simulink library "FlexBeamElement_MS2G_Lib"  (R2016a)
settings: Solver=ode45  StartTime=0.0  StopTime=10.0  RelTol=1e-3
undefined symbols (not defined in the file): b, beam_length, beam_wall, beam_width, bending_stiffness, Damping, density, Extr_Data_Box, kbendingx, kbendingy, kelongz, ktwistz, matDamping, num_elem, numelem, rho, shearM, X, Y, youngsM, Z
libraries: sm_lib x335, nesl_utility x64, FlexBeamElement_MS2G_Lib x1
(part 2 of 10)

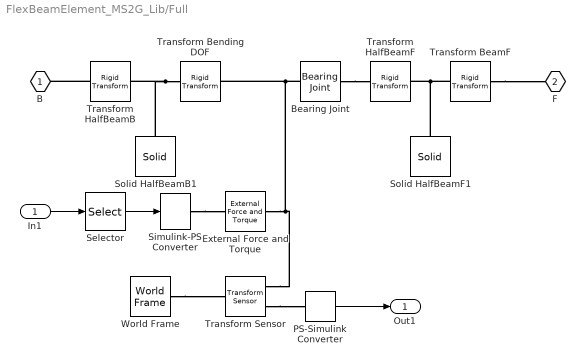
== system FlexBeamElement_MS2G_Lib/Full ==
  In1 : Inport
  " Transform Bending DOF" : sm_lib/Frames and Transforms/Rigid Transform  TranslationMethod=StandardAxis  TranslationLengthUnit=m  TranslationStandardAxis=+Z  TranslationStandardOffset=length/4  TranslationCartesianOffset=[0 0 0]  TranslationROffset=0  TranslationROffsetUnits=m  TranslationZOffset=0  TranslationZOffsetUnits=m  TranslationThetaOffset=0  TranslationThetaOffsetUnits=deg  RotationMethod=None  RotationAngleUnits=deg  RotationStandardAxis=+Y  RotationAngle=90  RotationArbitraryAxis=[0 0 1]  FollAlignAxisA=+X  BaseAlignAxisA=+Y  FollAlignAxisB=+Y  BaseAlignAxisB=+Z  RotationSequenceAxes=FollowerAxes  RotationSequence=XYX  RotationSequenceAngles=[0 0 0]  RotationSequenceAnglesUnits=deg  RotationMatrix=[1 0 0; 0 1 0; 0 0 1]
  " Transform BeamF" : sm_lib/Frames and Transforms/Rigid Transform  TranslationMethod=StandardAxis  TranslationLengthUnit=m  TranslationStandardAxis=+Z  TranslationStandardOffset=length/4  TranslationCartesianOffset=[0 0 0]  TranslationROffset=0  TranslationROffsetUnits=m  TranslationZOffset=0  TranslationZOffsetUnits=m  TranslationThetaOffset=0  TranslationThetaOffsetUnits=deg  RotationMethod=None  RotationAngleUnits=deg  RotationStandardAxis=+Z  RotationAngle=0  RotationArbitraryAxis=[0 0 1]  FollAlignAxisA=+X  BaseAlignAxisA=+Y  FollAlignAxisB=+Y  BaseAlignAxisB=+Z  RotationSequenceAxes=FollowerAxes  RotationSequence=XYX  RotationSequenceAngles=[0 0 0]  RotationSequenceAnglesUnits=deg  RotationMatrix=[1 0 0; 0 1 0; 0 0 1]
  Bearing Joint : sm_lib/Joints/Bearing Joint  SenseConstraintForce=off  SenseConstraintForceX=off  SenseConstraintForceY=off  SenseConstraintForceZ=off  SenseConstraintTorque=off  SenseConstraintTorqueX=off  SenseConstraintTorqueY=off  SenseConstraintTorqueZ=off  SenseTotalForce=off  SenseTotalForceX=off  SenseTotalForceY=off  SenseTotalForceZ=off  SenseTotalTorque=off  SenseTotalTorqueX=off  SenseTotalTorqueY=off  SenseTotalTorqueZ=off  CompositeWrenchDir=FollowerOnBase  CompositeWrenchFrame=BaseFrame  PzEquilibriumPosition=0  PzEquilibriumPositionUnits=m  PzSpringStiffness=kelongz  PzSpringStiffnessUnits=N/m  PzDampingCoefficient=b  PzDampingCoefficientUnits=N/(m/s)  PzTorqueActuationMode=NoTorque  PzMotionActuationMode=ComputedMotion  PzSensePosition=off  PzSenseVelocity=off  PzSenseAcceleration=off  PzSenseTorqueForce=off  PzPositionTargetSpecify=off  PzPositionTargetPriority=High  PzPositionTargetValue=0  PzPositionTargetValueUnits=m  PzVelocityTargetSpecify=off  PzVelocityTargetPriority=High  PzVelocityTargetValue=0  PzVelocityTargetValueUnits=m/s  RxEquilibriumPosition=0  RxEquilibriumPositionUnits=deg  RxSpringStiffness=kbendingx  RxSpringStiffnessUnits=N*m/rad  RxDampingCoefficient=b  RxDampingCoefficientUnits=N*m/(rad/s)  RxTorqueActuationMode=NoTorque  RxMotionActuationMode=ComputedMotion  RxSensePosition=off  RxSenseVelocity=off  RxSenseAcceleration=off  RxSenseTorqueForce=off  RxPositionTargetSpecify=off  RxPositionTargetPriority=High  RxPositionTargetValue=0  RxPositionTargetValueUnits=deg  RxVelocityTargetSpecify=off  RxVelocityTargetPriority=High  RxVelocityTargetValue=0  RxVelocityTargetValueUnits=deg/s  RyEquilibriumPosition=0  RyEquilibriumPositionUnits=deg  RySpringStiffness=kbendingy  RySpringStiffnessUnits=N*m/rad  RyDampingCoefficient=b  RyDampingCoefficientUnits=N*m/(rad/s)  RyTorqueActuationMode=NoTorque  RyMotionActuationMode=ComputedMotion  RySensePosition=off  RySenseVelocity=off  RySenseAcceleration=off  RySenseTorqueForce=off  RyPositionTargetSpecify=off  RyPositionTargetPriority=High  RyPositionTargetValue=0  RyPositionTargetValueUnits=deg  RyVelocityTargetSpecify=off  RyVelocityTargetPriority=High  RyVelocityTargetValue=0  RyVelocityTargetValueUnits=deg/s  RzEquilibriumPosition=0  RzEquilibriumPositionUnits=deg  RzSpringStiffness=ktwistz  RzSpringStiffnessUnits=N*m/rad  RzDampingCoefficient=b  RzDampingCoefficientUnits=N*m/(rad/s)  RzTorqueActuationMode=NoTorque  RzMotionActuationMode=ComputedMotion  RzSensePosition=off  RzSenseVelocity=off  RzSenseAcceleration=off  RzSenseTorqueForce=off  RzPositionTargetSpecify=off  RzPositionTargetPriority=High  RzPositionTargetValue=0  RzPositionTargetValueUnits=deg  RzVelocityTargetSpecify=off  RzVelocityTargetPriority=High  RzVelocityTargetValue=0  RzVelocityTargetValueUnits=deg/s
  External Force and Torque : sm_lib/Forces and Torques/External Force and Torque  ForceResolutionFrame=AttachedFrame  EnableForceX=off  EnableForceY=off  EnableForceZ=off  EnableForce=on  TorqueResolutionFrame=AttachedFrame  EnableTorqueX=off  EnableTorqueY=off  EnableTorqueZ=off  EnableTorque=off
  PS-Simulink Converter : nesl_utility/PS-Simulink Converter  PhysicalDomain=network_engine_domain  SubClassName=ps_output  LeftPortType=input  RightPortType=output  PseudoPeriodic=off  Frequencies=[]  Unit=1  AffineConversion=off
  Selector : Selector  InputPortWidth=numelem*3  IndexOptions=Index vector (dialog)  Indices=[1 3]  OutputSizes=1
  Simulink-PS Converter : nesl_utility/Simulink-PS Converter  PhysicalDomain=network_engine_domain  SubClassName=ps_input  LeftPortType=input  RightPortType=output  PseudoPeriodic=off  Frequencies=[]  NoiseDistribution=none  NoiseParameters=[]  Unit=1  AffineConversion=off  InputFiltering=off  SimscapeFilterOrder=1  InputFilterTimeConstant=0.001  UdotUserProvided=1
  Solid HalfBeamB1 : sm_lib/Body Elements/Solid  InertiaType=CalculateFromGeometry  Mass=1  MassUnits=kg  CenterOfMass=[0 0 0]  CenterOfMassUnits=m  MomentsOfInertia=[1 1 1]  MomentsOfInertiaUnits=kg*m^2  ProductsOfInertia=[0 0 0]  ProductsOfInertiaUnits=kg*m^2  DensityBased=on  Density=rho  DensityUnits=kg/(m^3)  DoExposeReferenceFrame=on  SerializedFrames=<Frames/>  GraphicType=FromGeometry  MarkerShape=Sphere  MarkerSize=10  MarkerSizeUnits=m  GraphicVisPropType=SimpleVisualProperties  GraphicDiffuseColor=[0.5 0.5 0.5]  GraphicSpecularColor=[0.5 0.5 0.5 1.0]  GraphicAmbientColor=[0.15 0.15 0.15 1.0]  GraphicEmissiveColor=[0.0 0.0 0.0 1.0]  GraphicShininess=75  GraphicOpacity=1.0  GeometryShape=GeneralExtrusion  RectangleSize=[1 1]  RectangleSizeUnits=m  BrickDimensions=[1 1 1]  BrickDimensionUnits=m  CylinderRadius=1  CylinderRadiusUnits=m  CylinderLength=1  CylinderLengthUnits=m  SphereRadius=1  SphereRadiusUnits=m  EllipsoidRadii=[1 1 1]  EllipsoidRadiiUnits=m  ExtrusionCrossSection=Extr_Data_Box(beam_width,beam_width-2*beam_wall,beam_width,beam_width-2*beam_wall)  ExtrusionCrossSectionUnits=m  ExtrusionLength=length/2  ExtrusionLengthUnits=m  PolygonNumSides=3  PolygonOuterRadius=1  PolygonOuterRadiusUnits=m  ExtGeomFileType=STL  ExtGeomFileUnits=m  RevolutionCrossSection=[1 1; 1 -1; 2 -1; 2 1]  RevolutionCrossSectionUnits=m  RevolutionExtent=Full  RevolutionAngle=180  RevolutionAngleUnits=deg
  Solid HalfBeamF1 : sm_lib/Body Elements/Solid  InertiaType=CalculateFromGeometry  Mass=1  MassUnits=kg  CenterOfMass=[0 0 0]  CenterOfMassUnits=m  MomentsOfInertia=[1 1 1]  MomentsOfInertiaUnits=kg*m^2  ProductsOfInertia=[0 0 0]  ProductsOfInertiaUnits=kg*m^2  DensityBased=on  Density=rho  DensityUnits=kg/(m^3)  DoExposeReferenceFrame=on  SerializedFrames=<Frames/>  GraphicType=FromGeometry  MarkerShape=Sphere  MarkerSize=10  MarkerSizeUnits=m  GraphicVisPropType=SimpleVisualProperties  GraphicDiffuseColor=[0.5 0.5 0.5]  GraphicSpecularColor=[0.5 0.5 0.5 1.0]  GraphicAmbientColor=[0.15 0.15 0.15 1.0]  GraphicEmissiveColor=[0.0 0.0 0.0 1.0]  GraphicShininess=75  GraphicOpacity=1.0  GeometryShape=GeneralExtrusion  RectangleSize=[1 1]  RectangleSizeUnits=m  BrickDimensions=[1 1 1]  BrickDimensionUnits=m  CylinderRadius=1  CylinderRadiusUnits=m  CylinderLength=1  CylinderLengthUnits=m  SphereRadius=1  SphereRadiusUnits=m  EllipsoidRadii=[1 1 1]  EllipsoidRadiiUnits=m  ExtrusionCrossSection=Extr_Data_Box(beam_width,beam_width-2*beam_wall,beam_width,beam_width-2*beam_wall)  ExtrusionCrossSectionUnits=m  ExtrusionLength=length/2  ExtrusionLengthUnits=m  PolygonNumSides=3  PolygonOuterRadius=1  PolygonOuterRadiusUnits=m  ExtGeomFileType=STL  ExtGeomFileUnits=m  RevolutionCrossSection=[1 1; 1 -1; 2 -1; 2 1]  RevolutionCrossSectionUnits=m  RevolutionExtent=Full  RevolutionAngle=180  RevolutionAngleUnits=deg
  Transform HalfBeamB : sm_lib/Frames and Transforms/Rigid Transform  TranslationMethod=StandardAxis  TranslationLengthUnit=m  TranslationStandardAxis=+Z  TranslationStandardOffset=length/4  TranslationCartesianOffset=[0 0 0]  TranslationROffset=0  TranslationROffsetUnits=m  TranslationZOffset=0  TranslationZOffsetUnits=m  TranslationThetaOffset=0  TranslationThetaOffsetUnits=deg  RotationMethod=None  RotationAngleUnits=deg  RotationStandardAxis=+Z  RotationAngle=0  RotationArbitraryAxis=[0 0 1]  FollAlignAxisA=+X  BaseAlignAxisA=+Y  FollAlignAxisB=+Y  BaseAlignAxisB=+Z  RotationSequenceAxes=FollowerAxes  RotationSequence=XYX  RotationSequenceAngles=[0 0 0]  RotationSequenceAnglesUnits=deg  RotationMatrix=[1 0 0; 0 1 0; 0 0 1]
  Transform HalfBeamF : sm_lib/Frames and Transforms/Rigid Transform  TranslationMethod=StandardAxis  TranslationLengthUnit=m  TranslationStandardAxis=+Z  TranslationStandardOffset=-length/4  TranslationCartesianOffset=[0 0 0]  TranslationROffset=0  TranslationROffsetUnits=m  TranslationZOffset=0  TranslationZOffsetUnits=m  TranslationThetaOffset=0  TranslationThetaOffsetUnits=deg  RotationMethod=None  RotationAngleUnits=deg  RotationStandardAxis=+Y  RotationAngle=90  RotationArbitraryAxis=[0 0 1]  FollAlignAxisA=+X  BaseAlignAxisA=+Y  FollAlignAxisB=+Y  BaseAlignAxisB=+Z  RotationSequenceAxes=FollowerAxes  RotationSequence=XYX  RotationSequenceAngles=[0 0 0]  RotationSequenceAnglesUnits=deg  RotationMatrix=[1 0 0; 0 1 0; 0 0 1]
  Transform Sensor : sm_lib/Frames and Transforms/Transform Sensor  MeasurementFrame=World  SenseAngle=off  SenseAxis=off  SenseAngle1=off  SenseAngle2=off  SenseAngle3=off  SenseQ=off  SenseR=off  SenseOmegaX=off  SenseOmegaY=off  SenseOmegaZ=on  SenseOmega1=off  SenseOmega2=off  SenseOmega3=off  SenseQDot=off  SenseRDot=off  SenseAlphaX=off  SenseAlphaY=off  SenseAlphaZ=off  SenseAlpha1=off  SenseAlpha2=off  SenseAlpha3=off  SenseQDDot=off  SenseRDDot=off  SenseX=off  SenseY=off  SenseZ=off  SenseRad=off  SenseAzim=off  SenseDist=off  SenseInc=off  SenseXDot=off  SenseYDot=off  SenseZDot=off  SenseRadDot=off  SenseAzimDot=off  SenseDistDot=off  SenseIncDot=off  SenseXDDot=off  SenseYDDot=off  SenseZDDot=off  SenseRadDDot=off  SenseAzimDDot=off  SenseDistDDot=off  SenseIncDDot=off
  World Frame : sm_lib/Frames and Transforms/World Frame
  B : PMIOPort  Port=1  Side=Left
  F : PMIOPort  Port=2  Side=Right
  Out1 : Outport
  wires:
  In1/1 -> Selector/1
  Selector/1 -> Simulink-PS Converter/1
  PS-Simulink Converter/1 -> Out1/1
  connections:
  External Force and Torque/RConn1 -- Transform Sensor/RConn1 -- " Transform Bending DOF"/RConn1 -- Bearing Joint/LConn1
  Bearing Joint/RConn1 -- Transform HalfBeamF/RConn1
  " Transform Bending DOF"/LConn1 -- Transform HalfBeamB/RConn1 -- Solid HalfBeamB1/RConn1
  Solid HalfBeamF1/RConn1 -- " Transform BeamF"/LConn1 -- Transform HalfBeamF/LConn1
  Transform HalfBeamB/LConn1 -- B/RConn1
  " Transform BeamF"/RConn1 -- F/RConn1
  Simulink-PS Converter/RConn1 -- External Force and Torque/LConn1
  World Frame/RConn1 -- Transform Sensor/LConn1
  Transform Sensor/RConn2 -- PS-Simulink Converter/LConn1

== system FlexBeamElement_MS2G_Lib/Flex_Body/Flex_Elem_1 ==
  In1 : Inport
  Full : Subsystem  mask{length=length, rho=rho, beam_width=beam_width, beam_wall=beam_wall, kbendingx=kbendingx, kbendingy=kbendingy, kbendingz=ktwistz, kelongz=kelongz, b=b}
      mask prompts: length "Beam Length (m)"; rho "Material Density (kg/(m^3)"; beam_width "Beam Width & Height (m)"; beam_wall "Beam Wall Thickness (m)"; kbendingx "Bending Spring Constant about X(Nm/rad)"; kbendingy "Bending Spring Constant about Y(Nm/rad)"; kbendingz "Twist Spring Constant about Z(Nm/rad)"; kelongz "Elongation Spring Constant about Z(N/m)"; b "Damping Constant (Nm/rad.s)"
  B : PMIOPort  Port=1  Side=Left
  F : PMIOPort  Port=2  Side=Right
  Out1 : Outport
  wires:
  In1/1 -> Full/1(In1)
  Full/1(Out1) -> Out1/1
  connections:
  Full/LConn1 -- B/RConn1
  Full/RConn1 -- F/RConn1

== system FlexBeamElement_MS2G_Lib/Flex_Body/Flex_Elem_10 ==
  In1 : Inport
  Full : Subsystem  mask{length=length, rho=rho, beam_width=beam_width, beam_wall=beam_wall, kbendingx=kbendingx, kbendingy=kbendingy, kbendingz=ktwistz, kelongz=kelongz, b=b}
      mask prompts: length "Beam Length (m)"; rho "Material Density (kg/(m^3)"; beam_width "Beam Width & Height (m)"; beam_wall "Beam Wall Thickness (m)"; kbendingx "Bending Spring Constant about X(Nm/rad)"; kbendingy "Bending Spring Constant about Y(Nm/rad)"; kbendingz "Twist Spring Constant about Z(Nm/rad)"; kelongz "Elongation Spring Constant about Z(N/m)"; b "Damping Constant (Nm/rad.s)"
  B : PMIOPort  Port=1  Side=Left
  F : PMIOPort  Port=2  Side=Right
  Out1 : Outport
  wires:
  In1/1 -> Full/1(In1)
  Full/1(Out1) -> Out1/1
  connections:
  Full/LConn1 -- B/RConn1
  Full/RConn1 -- F/RConn1

== system FlexBeamElement_MS2G_Lib/Flex_Body/Flex_Elem_11 ==
  In1 : Inport
  Full : Subsystem  mask{length=length, rho=rho, beam_width=beam_width, beam_wall=beam_wall, kbendingx=kbendingx, kbendingy=kbendingy, kbendingz=ktwistz, kelongz=kelongz, b=b}
      mask prompts: length "Beam Length (m)"; rho "Material Density (kg/(m^3)"; beam_width "Beam Width & Height (m)"; beam_wall "Beam Wall Thickness (m)"; kbendingx "Bending Spring Constant about X(Nm/rad)"; kbendingy "Bending Spring Constant about Y(Nm/rad)"; kbendingz "Twist Spring Constant about Z(Nm/rad)"; kelongz "Elongation Spring Constant about Z(N/m)"; b "Damping Constant (Nm/rad.s)"
  B : PMIOPort  Port=1  Side=Left
  F : PMIOPort  Port=2  Side=Right
  Out1 : Outport
  wires:
  In1/1 -> Full/1(In1)
  Full/1(Out1) -> Out1/1
  connections:
  Full/LConn1 -- B/RConn1
  Full/RConn1 -- F/RConn1

== system FlexBeamElement_MS2G_Lib/Flex_Body/Flex_Elem_12 ==
  In1 : Inport
  Full : Subsystem  mask{length=length, rho=rho, beam_width=beam_width, beam_wall=beam_wall, kbendingx=kbendingx, kbendingy=kbendingy, kbendingz=ktwistz, kelongz=kelongz, b=b}
      mask prompts: length "Beam Length (m)"; rho "Material Density (kg/(m^3)"; beam_width "Beam Width & Height (m)"; beam_wall "Beam Wall Thickness (m)"; kbendingx "Bending Spring Constant about X(Nm/rad)"; kbendingy "Bending Spring Constant about Y(Nm/rad)"; kbendingz "Twist Spring Constant about Z(Nm/rad)"; kelongz "Elongation Spring Constant about Z(N/m)"; b "Damping Constant (Nm/rad.s)"
  B : PMIOPort  Port=1  Side=Left
  F : PMIOPort  Port=2  Side=Right
  Out1 : Outport
  wires:
  In1/1 -> Full/1(In1)
  Full/1(Out1) -> Out1/1
  connections:
  Full/LConn1 -- B/RConn1
  Full/RConn1 -- F/RConn1

== system FlexBeamElement_MS2G_Lib/Flex_Body/Flex_Elem_13 ==
  In1 : Inport
  Full : Subsystem  mask{length=length, rho=rho, beam_width=beam_width, beam_wall=beam_wall, kbendingx=kbendingx, kbendingy=kbendingy, kbendingz=ktwistz, kelongz=kelongz, b=b}
      mask prompts: length "Beam Length (m)"; rho "Material Density (kg/(m^3)"; beam_width "Beam Width & Height (m)"; beam_wall "Beam Wall Thickness (m)"; kbendingx "Bending Spring Constant about X(Nm/rad)"; kbendingy "Bending Spring Constant about Y(Nm/rad)"; kbendingz "Twist Spring Constant about Z(Nm/rad)"; kelongz "Elongation Spring Constant about Z(N/m)"; b "Damping Constant (Nm/rad.s)"
  B : PMIOPort  Port=1  Side=Left
  F : PMIOPort  Port=2  Side=Right
  Out1 : Outport
  wires:
  In1/1 -> Full/1(In1)
  Full/1(Out1) -> Out1/1
  connections:
  Full/LConn1 -- B/RConn1
  Full/RConn1 -- F/RConn1

== system FlexBeamElement_MS2G_Lib/Flex_Body/Flex_Elem_14 ==
  In1 : Inport
  Full : Subsystem  mask{length=length, rho=rho, beam_width=beam_width, beam_wall=beam_wall, kbendingx=kbendingx, kbendingy=kbendingy, kbendingz=ktwistz, kelongz=kelongz, b=b}
      mask prompts: length "Beam Length (m)"; rho "Material Density (kg/(m^3)"; beam_width "Beam Width & Height (m)"; beam_wall "Beam Wall Thickness (m)"; kbendingx "Bending Spring Constant about X(Nm/rad)"; kbendingy "Bending Spring Constant about Y(Nm/rad)"; kbendingz "Twist Spring Constant about Z(Nm/rad)"; kelongz "Elongation Spring Constant about Z(N/m)"; b "Damping Constant (Nm/rad.s)"
  B : PMIOPort  Port=1  Side=Left
  F : PMIOPort  Port=2  Side=Right
  Out1 : Outport
  wires:
  In1/1 -> Full/1(In1)
  Full/1(Out1) -> Out1/1
  connections:
  Full/LConn1 -- B/RConn1
  Full/RConn1 -- F/RConn1

== system FlexBeamElement_MS2G_Lib/Flex_Body/Flex_Elem_15 ==
  In1 : Inport
  Full : Subsystem  mask{length=length, rho=rho, beam_width=beam_width, beam_wall=beam_wall, kbendingx=kbendingx, kbendingy=kbendingy, kbendingz=ktwistz, kelongz=kelongz, b=b}
      mask prompts: length "Beam Length (m)"; rho "Material Density (kg/(m^3)"; beam_width "Beam Width & Height (m)"; beam_wall "Beam Wall Thickness (m)"; kbendingx "Bending Spring Constant about X(Nm/rad)"; kbendingy "Bending Spring Constant about Y(Nm/rad)"; kbendingz "Twist Spring Constant about Z(Nm/rad)"; kelongz "Elongation Spring Constant about Z(N/m)"; b "Damping Constant (Nm/rad.s)"
  B : PMIOPort  Port=1  Side=Left
  F : PMIOPort  Port=2  Side=Right
  Out1 : Outport
  wires:
  In1/1 -> Full/1(In1)
  Full/1(Out1) -> Out1/1
  connections:
  Full/LConn1 -- B/RConn1
  Full/RConn1 -- F/RConn1

== system FlexBeamElement_MS2G_Lib/Flex_Body/Flex_Elem_16 ==
  In1 : Inport
  Full : Subsystem  mask{length=length, rho=rho, beam_width=beam_width, beam_wall=beam_wall, kbendingx=kbendingx, kbendingy=kbendingy, kbendingz=ktwistz, kelongz=kelongz, b=b}
      mask prompts: length "Beam Length (m)"; rho "Material Density (kg/(m^3)"; beam_width "Beam Width & Height (m)"; beam_wall "Beam Wall Thickness (m)"; kbendingx "Bending Spring Constant about X(Nm/rad)"; kbendingy "Bending Spring Constant about Y(Nm/rad)"; kbendingz "Twist Spring Constant about Z(Nm/rad)"; kelongz "Elongation Spring Constant about Z(N/m)"; b "Damping Constant (Nm/rad.s)"
  B : PMIOPort  Port=1  Side=Left
  F : PMIOPort  Port=2  Side=Right
  Out1 : Outport
  wires:
  In1/1 -> Full/1(In1)
  Full/1(Out1) -> Out1/1
  connections:
  Full/LConn1 -- B/RConn1
  Full/RConn1 -- F/RConn1

== system FlexBeamElement_MS2G_Lib/Flex_Body/Flex_Elem_17 ==
  In1 : Inport
  Full : Subsystem  mask{length=length, rho=rho, beam_width=beam_width, beam_wall=beam_wall, kbendingx=kbendingx, kbendingy=kbendingy, kbendingz=ktwistz, kelongz=kelongz, b=b}
      mask prompts: length "Beam Length (m)"; rho "Material Density (kg/(m^3)"; beam_width "Beam Width & Height (m)"; beam_wall "Beam Wall Thickness (m)"; kbendingx "Bending Spring Constant about X(Nm/rad)"; kbendingy "Bending Spring Constant about Y(Nm/rad)"; kbendingz "Twist Spring Constant about Z(Nm/rad)"; kelongz "Elongation Spring Constant about Z(N/m)"; b "Damping Constant (Nm/rad.s)"
  B : PMIOPort  Port=1  Side=Left
  F : PMIOPort  Port=2  Side=Right
  Out1 : Outport
  wires:
  In1/1 -> Full/1(In1)
  Full/1(Out1) -> Out1/1
  connections:
  Full/LConn1 -- B/RConn1
  Full/RConn1 -- F/RConn1

== system FlexBeamElement_MS2G_Lib/Flex_Body/Flex_Elem_18 ==
  In1 : Inport
  Full : Subsystem  mask{length=length, rho=rho, beam_width=beam_width, beam_wall=beam_wall, kbendingx=kbendingx, kbendingy=kbendingy, kbendingz=ktwistz, kelongz=kelongz, b=b}
      mask prompts: length "Beam Length (m)"; rho "Material Density (kg/(m^3)"; beam_width "Beam Width & Height (m)"; beam_wall "Beam Wall Thickness (m)"; kbendingx "Bending Spring Constant about X(Nm/rad)"; kbendingy "Bending Spring Constant about Y(Nm/rad)"; kbendingz "Twist Spring Constant about Z(Nm/rad)"; kelongz "Elongation Spring Constant about Z(N/m)"; b "Damping Constant (Nm/rad.s)"
  B : PMIOPort  Port=1  Side=Left
  F : PMIOPort  Port=2  Side=Right
  Out1 : Outport
  wires:
  In1/1 -> Full/1(In1)
  Full/1(Out1) -> Out1/1
  connections:
  Full/LConn1 -- B/RConn1
  Full/RConn1 -- F/RConn1

== system FlexBeamElement_MS2G_Lib/Flex_Body/Flex_Elem_19 ==
  In1 : Inport
  Full : Subsystem  mask{length=length, rho=rho, beam_width=beam_width, beam_wall=beam_wall, kbendingx=kbendingx, kbendingy=kbendingy, kbendingz=ktwistz, kelongz=kelongz, b=b}
      mask prompts: length "Beam Length (m)"; rho "Material Density (kg/(m^3)"; beam_width "Beam Width & Height (m)"; beam_wall "Beam Wall Thickness (m)"; kbendingx "Bending Spring Constant about X(Nm/rad)"; kbendingy "Bending Spring Constant about Y(Nm/rad)"; kbendingz "Twist Spring Constant about Z(Nm/rad)"; kelongz "Elongation Spring Constant about Z(N/m)"; b "Damping Constant (Nm/rad.s)"
  B : PMIOPort  Port=1  Side=Left
  F : PMIOPort  Port=2  Side=Right
  Out1 : Outport
  wires:
  In1/1 -> Full/1(In1)
  Full/1(Out1) -> Out1/1
  connections:
  Full/LConn1 -- B/RConn1
  Full/RConn1 -- F/RConn1

== system FlexBeamElement_MS2G_Lib/Flex_Body/Flex_Elem_2 ==
  In1 : Inport
  Full : Subsystem  mask{length=length, rho=rho, beam_width=beam_width, beam_wall=beam_wall, kbendingx=kbendingx, kbendingy=kbendingy, kbendingz=ktwistz, kelongz=kelongz, b=b}
      mask prompts: length "Beam Length (m)"; rho "Material Density (kg/(m^3)"; beam_width "Beam Width & Height (m)"; beam_wall "Beam Wall Thickness (m)"; kbendingx "Bending Spring Constant about X(Nm/rad)"; kbendingy "Bending Spring Constant about Y(Nm/rad)"; kbendingz "Twist Spring Constant about Z(Nm/rad)"; kelongz "Elongation Spring Constant about Z(N/m)"; b "Damping Constant (Nm/rad.s)"
  B : PMIOPort  Port=1  Side=Left
  F : PMIOPort  Port=2  Side=Right
  Out1 : Outport
  wires:
  In1/1 -> Full/1(In1)
  Full/1(Out1) -> Out1/1
  connections:
  Full/LConn1 -- B/RConn1
  Full/RConn1 -- F/RConn1

== system FlexBeamElement_MS2G_Lib/Flex_Body/Flex_Elem_20 ==
  In1 : Inport
  Full : Subsystem  mask{length=length, rho=rho, beam_width=beam_width, beam_wall=beam_wall, kbendingx=kbendingx, kbendingy=kbendingy, kbendingz=ktwistz, kelongz=kelongz, b=b}
      mask prompts: length "Beam Length (m)"; rho "Material Density (kg/(m^3)"; beam_width "Beam Width & Height (m)"; beam_wall "Beam Wall Thickness (m)"; kbendingx "Bending Spring Constant about X(Nm/rad)"; kbendingy "Bending Spring Constant about Y(Nm/rad)"; kbendingz "Twist Spring Constant about Z(Nm/rad)"; kelongz "Elongation Spring Constant about Z(N/m)"; b "Damping Constant (Nm/rad.s)"
  B : PMIOPort  Port=1  Side=Left
  F : PMIOPort  Port=2  Side=Right
  Out1 : Outport
  wires:
  In1/1 -> Full/1(In1)
  Full/1(Out1) -> Out1/1
  connections:
  Full/LConn1 -- B/RConn1
  Full/RConn1 -- F/RConn1

== system FlexBeamElement_MS2G_Lib/Flex_Body/Flex_Elem_21 ==
  In1 : Inport
  Full : Subsystem  mask{length=length, rho=rho, beam_width=beam_width, beam_wall=beam_wall, kbendingx=kbendingx, kbendingy=kbendingy, kbendingz=ktwistz, kelongz=kelongz, b=b}
      mask prompts: length "Beam Length (m)"; rho "Material Density (kg/(m^3)"; beam_width "Beam Width & Height (m)"; beam_wall "Beam Wall Thickness (m)"; kbendingx "Bending Spring Constant about X(Nm/rad)"; kbendingy "Bending Spring Constant about Y(Nm/rad)"; kbendingz "Twist Spring Constant about Z(Nm/rad)"; kelongz "Elongation Spring Constant about Z(N/m)"; b "Damping Constant (Nm/rad.s)"
  B : PMIOPort  Port=1  Side=Left
  F : PMIOPort  Port=2  Side=Right
  Out1 : Outport
  wires:
  In1/1 -> Full/1(In1)
  Full/1(Out1) -> Out1/1
  connections:
  Full/LConn1 -- B/RConn1
  Full/RConn1 -- F/RConn1

== system FlexBeamElement_MS2G_Lib/Flex_Body/Flex_Elem_22 ==
  In1 : Inport
  Full : Subsystem  mask{length=length, rho=rho, beam_width=beam_width, beam_wall=beam_wall, kbendingx=kbendingx, kbendingy=kbendingy, kbendingz=ktwistz, kelongz=kelongz, b=b}
      mask prompts: length "Beam Length (m)"; rho "Material Density (kg/(m^3)"; beam_width "Beam Width & Height (m)"; beam_wall "Beam Wall Thickness (m)"; kbendingx "Bending Spring Constant about X(Nm/rad)"; kbendingy "Bending Spring Constant about Y(Nm/rad)"; kbendingz "Twist Spring Constant about Z(Nm/rad)"; kelongz "Elongation Spring Constant about Z(N/m)"; b "Damping Constant (Nm/rad.s)"
  B : PMIOPort  Port=1  Side=Left
  F : PMIOPort  Port=2  Side=Right
  Out1 : Outport
  wires:
  In1/1 -> Full/1(In1)
  Full/1(Out1) -> Out1/1
  connections:
  Full/LConn1 -- B/RConn1
  Full/RConn1 -- F/RConn1

== system FlexBeamElement_MS2G_Lib/Flex_Body/Flex_Elem_23 ==
  In1 : Inport
  Full : Subsystem  mask{length=length, rho=rho, beam_width=beam_width, beam_wall=beam_wall, kbendingx=kbendingx, kbendingy=kbendingy, kbendingz=ktwistz, kelongz=kelongz, b=b}
      mask prompts: length "Beam Length (m)"; rho "Material Density (kg/(m^3)"; beam_width "Beam Width & Height (m)"; beam_wall "Beam Wall Thickness (m)"; kbendingx "Bending Spring Constant about X(Nm/rad)"; kbendingy "Bending Spring Constant about Y(Nm/rad)"; kbendingz "Twist Spring Constant about Z(Nm/rad)"; kelongz "Elongation Spring Constant about Z(N/m)"; b "Damping Constant (Nm/rad.s)"
  B : PMIOPort  Port=1  Side=Left
  F : PMIOPort  Port=2  Side=Right
  Out1 : Outport
  wires:
  In1/1 -> Full/1(In1)
  Full/1(Out1) -> Out1/1
  connections:
  Full/LConn1 -- B/RConn1
  Full/RConn1 -- F/RConn1

== system FlexBeamElement_MS2G_Lib/Flex_Body/Flex_Elem_24 ==
  In1 : Inport
  Full : Subsystem  mask{length=length, rho=rho, beam_width=beam_width, beam_wall=beam_wall, kbendingx=kbendingx, kbendingy=kbendingy, kbendingz=ktwistz, kelongz=kelongz, b=b}
      mask prompts: length "Beam Length (m)"; rho "Material Density (kg/(m^3)"; beam_width "Beam Width & Height (m)"; beam_wall "Beam Wall Thickness (m)"; kbendingx "Bending Spring Constant about X(Nm/rad)"; kbendingy "Bending Spring Constant about Y(Nm/rad)"; kbendingz "Twist Spring Constant about Z(Nm/rad)"; kelongz "Elongation Spring Constant about Z(N/m)"; b "Damping Constant (Nm/rad.s)"
  B : PMIOPort  Port=1  Side=Left
  F : PMIOPort  Port=2  Side=Right
  Out1 : Outport
  wires:
  In1/1 -> Full/1(In1)
  Full/1(Out1) -> Out1/1
  connections:
  Full/LConn1 -- B/RConn1
  Full/RConn1 -- F/RConn1

== system FlexBeamElement_MS2G_Lib/Flex_Body/Flex_Elem_25 ==
  In1 : Inport
  Full : Subsystem  mask{length=length, rho=rho, beam_width=beam_width, beam_wall=beam_wall, kbendingx=kbendingx, kbendingy=kbendingy, kbendingz=ktwistz, kelongz=kelongz, b=b}
      mask prompts: length "Beam Length (m)"; rho "Material Density (kg/(m^3)"; beam_width "Beam Width & Height (m)"; beam_wall "Beam Wall Thickness (m)"; kbendingx "Bending Spring Constant about X(Nm/rad)"; kbendingy "Bending Spring Constant about Y(Nm/rad)"; kbendingz "Twist Spring Constant about Z(Nm/rad)"; kelongz "Elongation Spring Constant about Z(N/m)"; b "Damping Constant (Nm/rad.s)"
  B : PMIOPort  Port=1  Side=Left
  F : PMIOPort  Port=2  Side=Right
  Out1 : Outport
  wires:
  In1/1 -> Full/1(In1)
  Full/1(Out1) -> Out1/1
  connections:
  Full/LConn1 -- B/RConn1
  Full/RConn1 -- F/RConn1

== system FlexBeamElement_MS2G_Lib/Flex_Body/Flex_Elem_26 ==
  In1 : Inport
  Full : Subsystem  mask{length=length, rho=rho, beam_width=beam_width, beam_wall=beam_wall, kbendingx=kbendingx, kbendingy=kbendingy, kbendingz=ktwistz, kelongz=kelongz, b=b}
      mask prompts: length "Beam Length (m)"; rho "Material Density (kg/(m^3)"; beam_width "Beam Width & Height (m)"; beam_wall "Beam Wall Thickness (m)"; kbendingx "Bending Spring Constant about X(Nm/rad)"; kbendingy "Bending Spring Constant about Y(Nm/rad)"; kbendingz "Twist Spring Constant about Z(Nm/rad)"; kelongz "Elongation Spring Constant about Z(N/m)"; b "Damping Constant (Nm/rad.s)"
  B : PMIOPort  Port=1  Side=Left
  F : PMIOPort  Port=2  Side=Right
  Out1 : Outport
  wires:
  In1/1 -> Full/1(In1)
  Full/1(Out1) -> Out1/1
  connections:
  Full/LConn1 -- B/RConn1
  Full/RConn1 -- F/RConn1

== system FlexBeamElement_MS2G_Lib/Flex_Body/Flex_Elem_27 ==
  In1 : Inport
  Full : Subsystem  mask{length=length, rho=rho, beam_width=beam_width, beam_wall=beam_wall, kbendingx=kbendingx, kbendingy=kbendingy, kbendingz=ktwistz, kelongz=kelongz, b=b}
      mask prompts: length "Beam Length (m)"; rho "Material Density (kg/(m^3)"; beam_width "Beam Width & Height (m)"; beam_wall "Beam Wall Thickness (m)"; kbendingx "Bending Spring Constant about X(Nm/rad)"; kbendingy "Bending Spring Constant about Y(Nm/rad)"; kbendingz "Twist Spring Constant about Z(Nm/rad)"; kelongz "Elongation Spring Constant about Z(N/m)"; b "Damping Constant (Nm/rad.s)"
  B : PMIOPort  Port=1  Side=Left
  F : PMIOPort  Port=2  Side=Right
  Out1 : Outport
  wires:
  In1/1 -> Full/1(In1)
  Full/1(Out1) -> Out1/1
  connections:
  Full/LConn1 -- B/RConn1
  Full/RConn1 -- F/RConn1

== system FlexBeamElement_MS2G_Lib/Flex_Body/Flex_Elem_28 ==
  In1 : Inport
  Full : Subsystem  mask{length=length, rho=rho, beam_width=beam_width, beam_wall=beam_wall, kbendingx=kbendingx, kbendingy=kbendingy, kbendingz=ktwistz, kelongz=kelongz, b=b}
      mask prompts: length "Beam Length (m)"; rho "Material Density (kg/(m^3)"; beam_width "Beam Width & Height (m)"; beam_wall "Beam Wall Thickness (m)"; kbendingx "Bending Spring Constant about X(Nm/rad)"; kbendingy "Bending Spring Constant about Y(Nm/rad)"; kbendingz "Twist Spring Constant about Z(Nm/rad)"; kelongz "Elongation Spring Constant about Z(N/m)"; b "Damping Constant (Nm/rad.s)"
  B : PMIOPort  Port=1  Side=Left
  F : PMIOPort  Port=2  Side=Right
  Out1 : Outport
  wires:
  In1/1 -> Full/1(In1)
  Full/1(Out1) -> Out1/1
  connections:
  Full/LConn1 -- B/RConn1
  Full/RConn1 -- F/RConn1

== system FlexBeamElement_MS2G_Lib/Flex_Body/Flex_Elem_29 ==
  In1 : Inport
  Full : Subsystem  mask{length=length, rho=rho, beam_width=beam_width, beam_wall=beam_wall, kbendingx=kbendingx, kbendingy=kbendingy, kbendingz=ktwistz, kelongz=kelongz, b=b}
      mask prompts: length "Beam Length (m)"; rho "Material Density (kg/(m^3)"; beam_width "Beam Width & Height (m)"; beam_wall "Beam Wall Thickness (m)"; kbendingx "Bending Spring Constant about X(Nm/rad)"; kbendingy "Bending Spring Constant about Y(Nm/rad)"; kbendingz "Twist Spring Constant about Z(Nm/rad)"; kelongz "Elongation Spring Constant about Z(N/m)"; b "Damping Constant (Nm/rad.s)"
  B : PMIOPort  Port=1  Side=Left
  F : PMIOPort  Port=2  Side=Right
  Out1 : Outport
  wires:
  In1/1 -> Full/1(In1)
  Full/1(Out1) -> Out1/1
  connections:
  Full/LConn1 -- B/RConn1
  Full/RConn1 -- F/RConn1

== system FlexBeamElement_MS2G_Lib/Flex_Body/Flex_Elem_3 ==
  In1 : Inport
  Full : Subsystem  mask{length=length, rho=rho, beam_width=beam_width, beam_wall=beam_wall, kbendingx=kbendingx, kbendingy=kbendingy, kbendingz=ktwistz, kelongz=kelongz, b=b}
      mask prompts: length "Beam Length (m)"; rho "Material Density (kg/(m^3)"; beam_width "Beam Width & Height (m)"; beam_wall "Beam Wall Thickness (m)"; kbendingx "Bending Spring Constant about X(Nm/rad)"; kbendingy "Bending Spring Constant about Y(Nm/rad)"; kbendingz "Twist Spring Constant about Z(Nm/rad)"; kelongz "Elongation Spring Constant about Z(N/m)"; b "Damping Constant (Nm/rad.s)"
  B : PMIOPort  Port=1  Side=Left
  F : PMIOPort  Port=2  Side=Right
  Out1 : Outport
  wires:
  In1/1 -> Full/1(In1)
  Full/1(Out1) -> Out1/1
  connections:
  Full/LConn1 -- B/RConn1
  Full/RConn1 -- F/RConn1

== system FlexBeamElement_MS2G_Lib/Flex_Body/Flex_Elem_30 ==
  In1 : Inport
  Full : Subsystem  mask{length=length, rho=rho, beam_width=beam_width, beam_wall=beam_wall, kbendingx=kbendingx, kbendingy=kbendingy, kbendingz=ktwistz, kelongz=kelongz, b=b}
      mask prompts: length "Beam Length (m)"; rho "Material Density (kg/(m^3)"; beam_width "Beam Width & Height (m)"; beam_wall "Beam Wall Thickness (m)"; kbendingx "Bending Spring Constant about X(Nm/rad)"; kbendingy "Bending Spring Constant about Y(Nm/rad)"; kbendingz "Twist Spring Constant about Z(Nm/rad)"; kelongz "Elongation Spring Constant about Z(N/m)"; b "Damping Constant (Nm/rad.s)"
  B : PMIOPort  Port=1  Side=Left
  F : PMIOPort  Port=2  Side=Right
  Out1 : Outport
  wires:
  In1/1 -> Full/1(In1)
  Full/1(Out1) -> Out1/1
  connections:
  Full/LConn1 -- B/RConn1
  Full/RConn1 -- F/RConn1

== system FlexBeamElement_MS2G_Lib/Flex_Body/Flex_Elem_4 ==
  In1 : Inport
  Full : Subsystem  mask{length=length, rho=rho, beam_width=beam_width, beam_wall=beam_wall, kbendingx=kbendingx, kbendingy=kbendingy, kbendingz=ktwistz, kelongz=kelongz, b=b}
      mask prompts: length "Beam Length (m)"; rho "Material Density (kg/(m^3)"; beam_width "Beam Width & Height (m)"; beam_wall "Beam Wall Thickness (m)"; kbendingx "Bending Spring Constant about X(Nm/rad)"; kbendingy "Bending Spring Constant about Y(Nm/rad)"; kbendingz "Twist Spring Constant about Z(Nm/rad)"; kelongz "Elongation Spring Constant about Z(N/m)"; b "Damping Constant (Nm/rad.s)"
  B : PMIOPort  Port=1  Side=Left
  F : PMIOPort  Port=2  Side=Right
  Out1 : Outport
  wires:
  In1/1 -> Full/1(In1)
  Full/1(Out1) -> Out1/1
  connections:
  Full/LConn1 -- B/RConn1
  Full/RConn1 -- F/RConn1

== system FlexBeamElement_MS2G_Lib/Flex_Body/Flex_Elem_5 ==
  In1 : Inport
  Full : Subsystem  mask{length=length, rho=rho, beam_width=beam_width, beam_wall=beam_wall, kbendingx=kbendingx, kbendingy=kbendingy, kbendingz=ktwistz, kelongz=kelongz, b=b}
      mask prompts: length "Beam Length (m)"; rho "Material Density (kg/(m^3)"; beam_width "Beam Width & Height (m)"; beam_wall "Beam Wall Thickness (m)"; kbendingx "Bending Spring Constant about X(Nm/rad)"; kbendingy "Bending Spring Constant about Y(Nm/rad)"; kbendingz "Twist Spring Constant about Z(Nm/rad)"; kelongz "Elongation Spring Constant about Z(N/m)"; b "Damping Constant (Nm/rad.s)"
  B : PMIOPort  Port=1  Side=Left
  F : PMIOPort  Port=2  Side=Right
  Out1 : Outport
  wires:
  In1/1 -> Full/1(In1)
  Full/1(Out1) -> Out1/1
  connections:
  Full/LConn1 -- B/RConn1
  Full/RConn1 -- F/RConn1

== system FlexBeamElement_MS2G_Lib/Flex_Body/Flex_Elem_6 ==
  In1 : Inport
  Full : Subsystem  mask{length=length, rho=rho, beam_width=beam_width, beam_wall=beam_wall, kbendingx=kbendingx, kbendingy=kbendingy, kbendingz=ktwistz, kelongz=kelongz, b=b}
      mask prompts: length "Beam Length (m)"; rho "Material Density (kg/(m^3)"; beam_width "Beam Width & Height (m)"; beam_wall "Beam Wall Thickness (m)"; kbendingx "Bending Spring Constant about X(Nm/rad)"; kbendingy "Bending Spring Constant about Y(Nm/rad)"; kbendingz "Twist Spring Constant about Z(Nm/rad)"; kelongz "Elongation Spring Constant about Z(N/m)"; b "Damping Constant (Nm/rad.s)"
  B : PMIOPort  Port=1  Side=Left
  F : PMIOPort  Port=2  Side=Right
  Out1 : Outport
  wires:
  In1/1 -> Full/1(In1)
  Full/1(Out1) -> Out1/1
  connections:
  Full/LConn1 -- B/RConn1
  Full/RConn1 -- F/RConn1

== system FlexBeamElement_MS2G_Lib/Flex_Body/Flex_Elem_7 ==
  In1 : Inport
  Full : Subsystem  mask{length=length, rho=rho, beam_width=beam_width, beam_wall=beam_wall, kbendingx=kbendingx, kbendingy=kbendingy, kbendingz=ktwistz, kelongz=kelongz, b=b}
      mask prompts: length "Beam Length (m)"; rho "Material Density (kg/(m^3)"; beam_width "Beam Width & Height (m)"; beam_wall "Beam Wall Thickness (m)"; kbendingx "Bending Spring Constant about X(Nm/rad)"; kbendingy "Bending Spring Constant about Y(Nm/rad)"; kbendingz "Twist Spring Constant about Z(Nm/rad)"; kelongz "Elongation Spring Constant about Z(N/m)"; b "Damping Constant (Nm/rad.s)"
  B : PMIOPort  Port=1  Side=Left
  F : PMIOPort  Port=2  Side=Right
  Out1 : Outport
  wires:
  In1/1 -> Full/1(In1)
  Full/1(Out1) -> Out1/1
  connections:
  Full/LConn1 -- B/RConn1
  Full/RConn1 -- F/RConn1

== system FlexBeamElement_MS2G_Lib/Flex_Body/Flex_Elem_8 ==
  In1 : Inport
  Full : Subsystem  mask{length=length, rho=rho, beam_width=beam_width, beam_wall=beam_wall, kbendingx=kbendingx, kbendingy=kbendingy, kbendingz=ktwistz, kelongz=kelongz, b=b}
      mask prompts: length "Beam Length (m)"; rho "Material Density (kg/(m^3)"; beam_width "Beam Width & Height (m)"; beam_wall "Beam Wall Thickness (m)"; kbendingx "Bending Spring Constant about X(Nm/rad)"; kbendingy "Bending Spring Constant about Y(Nm/rad)"; kbendingz "Twist Spring Constant about Z(Nm/rad)"; kelongz "Elongation Spring Constant about Z(N/m)"; b "Damping Constant (Nm/rad.s)"
  B : PMIOPort  Port=1  Side=Left
  F : PMIOPort  Port=2  Side=Right
  Out1 : Outport
  wires:
  In1/1 -> Full/1(In1)
  Full/1(Out1) -> Out1/1
  connections:
  Full/LConn1 -- B/RConn1
  Full/RConn1 -- F/RConn1

== system FlexBeamElement_MS2G_Lib/Flex_Body/Flex_Elem_9 ==
  In1 : Inport
  Full : Subsystem  mask{length=length, rho=rho, beam_width=beam_width, beam_wall=beam_wall, kbendingx=kbendingx, kbendingy=kbendingy, kbendingz=ktwistz, kelongz=kelongz, b=b}
      mask prompts: length "Beam Length (m)"; rho "Material Density (kg/(m^3)"; beam_width "Beam Width & Height (m)"; beam_wall "Beam Wall Thickness (m)"; kbendingx "Bending Spring Constant about X(Nm/rad)"; kbendingy "Bending Spring Constant about Y(Nm/rad)"; kbendingz "Twist Spring Constant about Z(Nm/rad)"; kelongz "Elongation Spring Constant about Z(N/m)"; b "Damping Constant (Nm/rad.s)"
  B : PMIOPort  Port=1  Side=Left
  F : PMIOPort  Port=2  Side=Right
  Out1 : Outport
  wires:
  In1/1 -> Full/1(In1)
  Full/1(Out1) -> Out1/1
  connections:
  Full/LConn1 -- B/RConn1
  Full/RConn1 -- F/RConn1

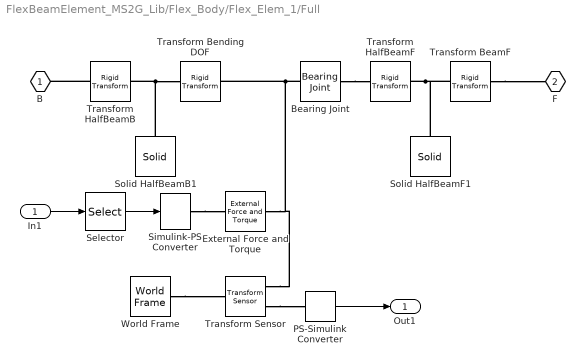
== system FlexBeamElement_MS2G_Lib/Flex_Body/Flex_Elem_1/Full ==
  In1 : Inport
  " Transform Bending DOF" : sm_lib/Frames and Transforms/Rigid Transform  TranslationMethod=StandardAxis  TranslationLengthUnit=m  TranslationStandardAxis=+Z  TranslationStandardOffset=length/4  TranslationCartesianOffset=[0 0 0]  TranslationROffset=0  TranslationROffsetUnits=m  TranslationZOffset=0  TranslationZOffsetUnits=m  TranslationThetaOffset=0  TranslationThetaOffsetUnits=deg  RotationMethod=None  RotationAngleUnits=deg  RotationStandardAxis=+Y  RotationAngle=90  RotationArbitraryAxis=[0 0 1]  FollAlignAxisA=+X  BaseAlignAxisA=+Y  FollAlignAxisB=+Y  BaseAlignAxisB=+Z  RotationSequenceAxes=FollowerAxes  RotationSequence=XYX  RotationSequenceAngles=[0 0 0]  RotationSequenceAnglesUnits=deg  RotationMatrix=[1 0 0; 0 1 0; 0 0 1]
  " Transform BeamF" : sm_lib/Frames and Transforms/Rigid Transform  TranslationMethod=StandardAxis  TranslationLengthUnit=m  TranslationStandardAxis=+Z  TranslationStandardOffset=length/4  TranslationCartesianOffset=[0 0 0]  TranslationROffset=0  TranslationROffsetUnits=m  TranslationZOffset=0  TranslationZOffsetUnits=m  TranslationThetaOffset=0  TranslationThetaOffsetUnits=deg  RotationMethod=None  RotationAngleUnits=deg  RotationStandardAxis=+Z  RotationAngle=0  RotationArbitraryAxis=[0 0 1]  FollAlignAxisA=+X  BaseAlignAxisA=+Y  FollAlignAxisB=+Y  BaseAlignAxisB=+Z  RotationSequenceAxes=FollowerAxes  RotationSequence=XYX  RotationSequenceAngles=[0 0 0]  RotationSequenceAnglesUnits=deg  RotationMatrix=[1 0 0; 0 1 0; 0 0 1]
  Bearing Joint : sm_lib/Joints/Bearing Joint  SenseConstraintForce=off  SenseConstraintForceX=off  SenseConstraintForceY=off  SenseConstraintForceZ=off  SenseConstraintTorque=off  SenseConstraintTorqueX=off  SenseConstraintTorqueY=off  SenseConstraintTorqueZ=off  SenseTotalForce=off  SenseTotalForceX=off  SenseTotalForceY=off  SenseTotalForceZ=off  SenseTotalTorque=off  SenseTotalTorqueX=off  SenseTotalTorqueY=off  SenseTotalTorqueZ=off  CompositeWrenchDir=FollowerOnBase  CompositeWrenchFrame=BaseFrame  PzEquilibriumPosition=0  PzEquilibriumPositionUnits=m  PzSpringStiffness=kelongz  PzSpringStiffnessUnits=N/m  PzDampingCoefficient=b  PzDampingCoefficientUnits=N/(m/s)  PzTorqueActuationMode=NoTorque  PzMotionActuationMode=ComputedMotion  PzSensePosition=off  PzSenseVelocity=off  PzSenseAcceleration=off  PzSenseTorqueForce=off  PzPositionTargetSpecify=off  PzPositionTargetPriority=High  PzPositionTargetValue=0  PzPositionTargetValueUnits=m  PzVelocityTargetSpecify=off  PzVelocityTargetPriority=High  PzVelocityTargetValue=0  PzVelocityTargetValueUnits=m/s  RxEquilibriumPosition=0  RxEquilibriumPositionUnits=deg  RxSpringStiffness=kbendingx  RxSpringStiffnessUnits=N*m/rad  RxDampingCoefficient=b  RxDampingCoefficientUnits=N*m/(rad/s)  RxTorqueActuationMode=NoTorque  RxMotionActuationMode=ComputedMotion  RxSensePosition=off  RxSenseVelocity=off  RxSenseAcceleration=off  RxSenseTorqueForce=off  RxPositionTargetSpecify=off  RxPositionTargetPriority=High  RxPositionTargetValue=0  RxPositionTargetValueUnits=deg  RxVelocityTargetSpecify=off  RxVelocityTargetPriority=High  RxVelocityTargetValue=0  RxVelocityTargetValueUnits=deg/s  RyEquilibriumPosition=0  RyEquilibriumPositionUnits=deg  RySpringStiffness=kbendingy  RySpringStiffnessUnits=N*m/rad  RyDampingCoefficient=b  RyDampingCoefficientUnits=N*m/(rad/s)  RyTorqueActuationMode=NoTorque  RyMotionActuationMode=ComputedMotion  RySensePosition=off  RySenseVelocity=off  RySenseAcceleration=off  RySenseTorqueForce=off  RyPositionTargetSpecify=off  RyPositionTargetPriority=High  RyPositionTargetValue=0  RyPositionTargetValueUnits=deg  RyVelocityTargetSpecify=off  RyVelocityTargetPriority=High  RyVelocityTargetValue=0  RyVelocityTargetValueUnits=deg/s  RzEquilibriumPosition=0  RzEquilibriumPositionUnits=deg  RzSpringStiffness=ktwistz  RzSpringStiffnessUnits=N*m/rad  RzDampingCoefficient=b  RzDampingCoefficientUnits=N*m/(rad/s)  RzTorqueActuationMode=NoTorque  RzMotionActuationMode=ComputedMotion  RzSensePosition=off  RzSenseVelocity=off  RzSenseAcceleration=off  RzSenseTorqueForce=off  RzPositionTargetSpecify=off  RzPositionTargetPriority=High  RzPositionTargetValue=0  RzPositionTargetValueUnits=deg  RzVelocityTargetSpecify=off  RzVelocityTargetPriority=High  RzVelocityTargetValue=0  RzVelocityTargetValueUnits=deg/s
  External Force and Torque : sm_lib/Forces and Torques/External Force and Torque  ForceResolutionFrame=AttachedFrame  EnableForceX=off  EnableForceY=off  EnableForceZ=off  EnableForce=on  TorqueResolutionFrame=AttachedFrame  EnableTorqueX=off  EnableTorqueY=off  EnableTorqueZ=off  EnableTorque=off
  PS-Simulink Converter : nesl_utility/PS-Simulink Converter  PhysicalDomain=network_engine_domain  SubClassName=ps_output  LeftPortType=input  RightPortType=output  PseudoPeriodic=off  Frequencies=[]  Unit=1  AffineConversion=off
  Selector : Selector  InputPortWidth=3*numelem  IndexOptions=Index vector (dialog)  Indices=[1 2 3]  OutputSizes=1
  Simulink-PS Converter : nesl_utility/Simulink-PS Converter  PhysicalDomain=network_engine_domain  SubClassName=ps_input  LeftPortType=input  RightPortType=output  PseudoPeriodic=off  Frequencies=[]  NoiseDistribution=none  NoiseParameters=[]  Unit=1  AffineConversion=off  InputFiltering=off  SimscapeFilterOrder=1  InputFilterTimeConstant=0.001  UdotUserProvided=1
  Solid HalfBeamB1 : sm_lib/Body Elements/Solid  InertiaType=CalculateFromGeometry  Mass=1  MassUnits=kg  CenterOfMass=[0 0 0]  CenterOfMassUnits=m  MomentsOfInertia=[1 1 1]  MomentsOfInertiaUnits=kg*m^2  ProductsOfInertia=[0 0 0]  ProductsOfInertiaUnits=kg*m^2  DensityBased=on  Density=rho  DensityUnits=kg/(m^3)  DoExposeReferenceFrame=on  SerializedFrames=<Frames/>  GraphicType=FromGeometry  MarkerShape=Sphere  MarkerSize=10  MarkerSizeUnits=m  GraphicVisPropType=SimpleVisualProperties  GraphicDiffuseColor=[0.5 0.5 0.5]  GraphicSpecularColor=[0.5 0.5 0.5 1.0]  GraphicAmbientColor=[0.15 0.15 0.15 1.0]  GraphicEmissiveColor=[0.0 0.0 0.0 1.0]  GraphicShininess=75  GraphicOpacity=1.0  GeometryShape=GeneralExtrusion  RectangleSize=[1 1]  RectangleSizeUnits=m  BrickDimensions=[1 1 1]  BrickDimensionUnits=m  CylinderRadius=1  CylinderRadiusUnits=m  CylinderLength=1  CylinderLengthUnits=m  SphereRadius=1  SphereRadiusUnits=m  EllipsoidRadii=[1 1 1]  EllipsoidRadiiUnits=m  ExtrusionCrossSection=Extr_Data_Box(beam_width,beam_width-2*beam_wall,beam_width,beam_width-2*beam_wall)  ExtrusionCrossSectionUnits=m  ExtrusionLength=length/2  ExtrusionLengthUnits=m  PolygonNumSides=3  PolygonOuterRadius=1  PolygonOuterRadiusUnits=m  ExtGeomFileType=STL  ExtGeomFileUnits=m  RevolutionCrossSection=[1 1; 1 -1; 2 -1; 2 1]  RevolutionCrossSectionUnits=m  RevolutionExtent=Full  RevolutionAngle=180  RevolutionAngleUnits=deg
  Solid HalfBeamF1 : sm_lib/Body Elements/Solid  InertiaType=CalculateFromGeometry  Mass=1  MassUnits=kg  CenterOfMass=[0 0 0]  CenterOfMassUnits=m  MomentsOfInertia=[1 1 1]  MomentsOfInertiaUnits=kg*m^2  ProductsOfInertia=[0 0 0]  ProductsOfInertiaUnits=kg*m^2  DensityBased=on  Density=rho  DensityUnits=kg/(m^3)  DoExposeReferenceFrame=on  SerializedFrames=<Frames/>  GraphicType=FromGeometry  MarkerShape=Sphere  MarkerSize=10  MarkerSizeUnits=m  GraphicVisPropType=SimpleVisualProperties  GraphicDiffuseColor=[0.5 0.5 0.5]  GraphicSpecularColor=[0.5 0.5 0.5 1.0]  GraphicAmbientColor=[0.15 0.15 0.15 1.0]  GraphicEmissiveColor=[0.0 0.0 0.0 1.0]  GraphicShininess=75  GraphicOpacity=1.0  GeometryShape=GeneralExtrusion  RectangleSize=[1 1]  RectangleSizeUnits=m  BrickDimensions=[1 1 1]  BrickDimensionUnits=m  CylinderRadius=1  CylinderRadiusUnits=m  CylinderLength=1  CylinderLengthUnits=m  SphereRadius=1  SphereRadiusUnits=m  EllipsoidRadii=[1 1 1]  EllipsoidRadiiUnits=m  ExtrusionCrossSection=Extr_Data_Box(beam_width,beam_width-2*beam_wall,beam_width,beam_width-2*beam_wall)  ExtrusionCrossSectionUnits=m  ExtrusionLength=length/2  ExtrusionLengthUnits=m  PolygonNumSides=3  PolygonOuterRadius=1  PolygonOuterRadiusUnits=m  ExtGeomFileType=STL  ExtGeomFileUnits=m  RevolutionCrossSection=[1 1; 1 -1; 2 -1; 2 1]  RevolutionCrossSectionUnits=m  RevolutionExtent=Full  RevolutionAngle=180  RevolutionAngleUnits=deg
  Transform HalfBeamB : sm_lib/Frames and Transforms/Rigid Transform  TranslationMethod=StandardAxis  TranslationLengthUnit=m  TranslationStandardAxis=+Z  TranslationStandardOffset=length/4  TranslationCartesianOffset=[0 0 0]  TranslationROffset=0  TranslationROffsetUnits=m  TranslationZOffset=0  TranslationZOffsetUnits=m  TranslationThetaOffset=0  TranslationThetaOffsetUnits=deg  RotationMethod=None  RotationAngleUnits=deg  RotationStandardAxis=+Z  RotationAngle=0  RotationArbitraryAxis=[0 0 1]  FollAlignAxisA=+X  BaseAlignAxisA=+Y  FollAlignAxisB=+Y  BaseAlignAxisB=+Z  RotationSequenceAxes=FollowerAxes  RotationSequence=XYX  RotationSequenceAngles=[0 0 0]  RotationSequenceAnglesUnits=deg  RotationMatrix=[1 0 0; 0 1 0; 0 0 1]
  Transform HalfBeamF : sm_lib/Frames and Transforms/Rigid Transform  TranslationMethod=StandardAxis  TranslationLengthUnit=m  TranslationStandardAxis=+Z  TranslationStandardOffset=-length/4  TranslationCartesianOffset=[0 0 0]  TranslationROffset=0  TranslationROffsetUnits=m  TranslationZOffset=0  TranslationZOffsetUnits=m  TranslationThetaOffset=0  TranslationThetaOffsetUnits=deg  RotationMethod=None  RotationAngleUnits=deg  RotationStandardAxis=+Y  RotationAngle=90  RotationArbitraryAxis=[0 0 1]  FollAlignAxisA=+X  BaseAlignAxisA=+Y  FollAlignAxisB=+Y  BaseAlignAxisB=+Z  RotationSequenceAxes=FollowerAxes  RotationSequence=XYX  RotationSequenceAngles=[0 0 0]  RotationSequenceAnglesUnits=deg  RotationMatrix=[1 0 0; 0 1 0; 0 0 1]
  Transform Sensor : sm_lib/Frames and Transforms/Transform Sensor  MeasurementFrame=World  SenseAngle=off  SenseAxis=off  SenseAngle1=off  SenseAngle2=off  SenseAngle3=off  SenseQ=off  SenseR=off  SenseOmegaX=off  SenseOmegaY=off  SenseOmegaZ=on  SenseOmega1=off  SenseOmega2=off  SenseOmega3=off  SenseQDot=off  SenseRDot=off  SenseAlphaX=off  SenseAlphaY=off  SenseAlphaZ=off  SenseAlpha1=off  SenseAlpha2=off  SenseAlpha3=off  SenseQDDot=off  SenseRDDot=off  SenseX=off  SenseY=off  SenseZ=off  SenseRad=off  SenseAzim=off  SenseDist=off  SenseInc=off  SenseXDot=off  SenseYDot=off  SenseZDot=off  SenseRadDot=off  SenseAzimDot=off  SenseDistDot=off  SenseIncDot=off  SenseXDDot=off  SenseYDDot=off  SenseZDDot=off  SenseRadDDot=off  SenseAzimDDot=off  SenseDistDDot=off  SenseIncDDot=off
  World Frame : sm_lib/Frames and Transforms/World Frame
  B : PMIOPort  Port=1  Side=Left
  F : PMIOPort  Port=2  Side=Right
  Out1 : Outport
  wires:
  PS-Simulink Converter/1 -> Out1/1
  Selector/1 -> Simulink-PS Converter/1
  In1/1 -> Selector/1
  connections:
  Transform Sensor/RConn2 -- PS-Simulink Converter/LConn1
  World Frame/RConn1 -- Transform Sensor/LConn1
  Simulink-PS Converter/RConn1 -- External Force and Torque/LConn1
  " Transform BeamF"/RConn1 -- F/RConn1
  Transform HalfBeamB/LConn1 -- B/RConn1
  Transform HalfBeamF/LConn1 -- " Transform BeamF"/LConn1 -- Solid HalfBeamF1/RConn1
  Solid HalfBeamB1/RConn1 -- Transform HalfBeamB/RConn1 -- " Transform Bending DOF"/LConn1
  Bearing Joint/RConn1 -- Transform HalfBeamF/RConn1
  Bearing Joint/LConn1 -- " Transform Bending DOF"/RConn1 -- Transform Sensor/RConn1 -- External Force and Torque/RConn1
